simulink model "CrazyClover_angular_velocity_control_PID"  (R2020b)
settings: Solver=VariableStepAuto  StartTime=0.0  StopTime=0.1  RelTol=1e-3
libraries: pid_lib x1
settings Model: Creator=kt012  LastModifiedBy=kt012

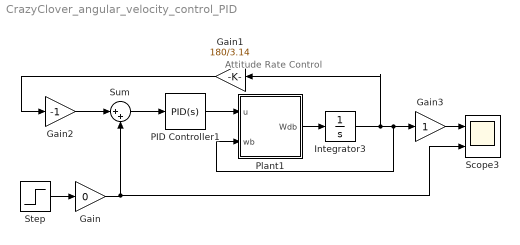
== system CrazyClover_angular_velocity_control_PID ==
  note: Attitude Rate Control
  Gain : Gain  Gain=0
  Gain1 : Gain  Gain=180/3.14
  Gain2 : Gain  Gain=-1
  Gain3 : Gain
  Integrator3 : Integrator  InitialCondition=[1 0 0];  ContinuousStateAttributes='Wb'
  PID Controller1 : pid_lib/PID Controller  Controller=PID  Form=Parallel  TimeDomain=Continuous-time  UseExternalTs=off  SampleTime=-1  IntegratorMethod=Forward Euler  FilterMethod=Forward Euler  ControllerParametersSource=internal  P=50  I=50  D=0  UseFilter=on  N=100  TunerSelectOption=Transfer Function Based (PID Tuner App)  InitialConditionSource=internal  InitialConditionForIntegrator=0  InitialConditionForFilter=0  DifferentiatorICPrevScaledInput=0  ExternalReset=none  TrackingMode=off  Kt=1  LimitOutput=off  SatLimitsSource=internal  UpperSaturationLimit=inf  LowerSaturationLimit=-inf  LinearizeAsGain=on  AntiWindupMode=none  Kb=1  POutMin=[]  POutMax=[]  IOutMin=[]  IOutMax=[]  DOutMin=[]  DOutMax=[]  NOutMin=[]  NOutMax=[]  SumOutMin=[]  SumOutMax=[]  SaturationOutMin=[]  SaturationOutMax=[]  PParamMin=[]  PParamMax=[]  IParamMin=[]  IParamMax=[]  DParamMin=[]  DParamMax=[]  NParamMin=[]  NParamMax=[]  KbParamMin=[]  KbParamMax=[]  KtParamMin=[]  KtParamMax=[]  KbOutMin=[]  KbOutMax=[]  KtOutMin=[]  KtOutMax=[]  IntegratorOutMin=[]  IntegratorOutMax=[]  FilterOutMin=[]  FilterOutMax=[]  SumI1OutMin=[]  SumI1OutMax=[]  SumI2OutMin=[]  SumI2OutMax=[]  SumI3OutMin=[]  SumI3OutMax=[]  SumI4OutMin=[]  SumI4OutMax=[]  SumDOutMin=[]  SumDOutMax=[]  DifferentiatorOutMin=[]  DifferentiatorOutMax=[]  FilterDiffOutCoefMin=[]  FilterDiffOutCoefMax=[]  ReciprocalOutMin=[]  ReciprocalOutMax=[]  SumDenOutMin=[]  SumDenOutMax=[]  SumNumOutMin=[]  SumNumOutMax=[]  DivideOutMin=[]  DivideOutMax=[]  UdiffTsProdOutMin=[]  UdiffTsProdOutMax=[]  NTsProdOutMin=[]  NTsProdOutMax=[]  UintegralTsProdOutMin=[]  UintegralTsProdOutMax=[]  UngainTsProdOutMin=[]  UngainTsProdOutMax=[]  IntegratorContinuousStateAttributes=''  IntegratorStateMustResolveToSignalObject=off  IntegratorRTWStateStorageClass=Auto  FilterContinuousStateAttributes=''  FilterStateMustResolveToSignalObject=off  FilterRTWStateStorageClass=Auto  ParallelPVariant=InternalParameters  IdealPVariant=Disabled  IVariant=InternalParameters  DVariant=InternalParameters  IntegratorVariant=Continuous  SatVariant=Disabled  AWVariant=Passthrough  PCopyVariant=Disabled  TRVariant=Disabled  FdbkBlocksVariant=Forward  IdealPFdbkVariant=Disabled  SatFdbkVariant=Disabled  DerivativeFilterVariant=ContFilter  NVariant=InternalParameters  NCopyVariant=Disabled  FilterICVariant=InternalICsFilter  IntegratorICVariant=InternalICs  ExternalResetVariant=Disabled  TRSumVariant=Passthrough  SumFdbkVariant=Disabled  SumVariant=Sum_PID  TsampFilterVariant=InternalTs  TsampNgainVariant=Passthrough  TsampIntegralVariant=Passthrough  ExternalSaturationOutDataTypeStr=Inherit: Same as second input
  Plant1 : Subsystem
  Scope3 : Scope  NumInputPorts=2
  Step : Step  Time=0.5  After=[1 0 0];  SampleTime=0
  Sum : Sum  Inputs=|++
  wires:
  PID Controller1/1 -> Plant1/1(u)
  Plant1/1(Wdb) -> Integrator3/1
  Sum/1 -> PID Controller1/1
  Gain2/1 -> Sum/1
  Integrator3/1 -> Gain1/1, Plant1/2(wb), Gain3/1
  Gain1/1 -> Gain2/1
  Step/1 -> Gain/1
  Gain3/1 -> Scope3/1
  Gain/1 -> Scope3/2, Sum/2

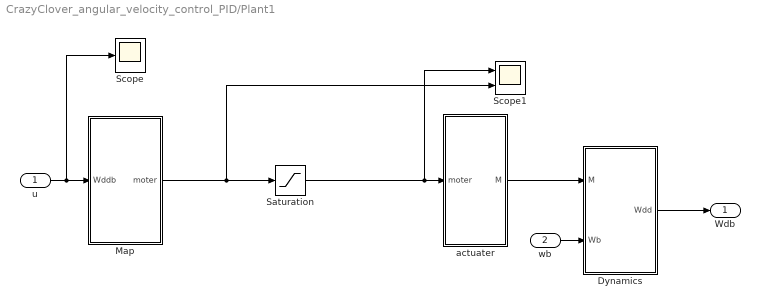
== system CrazyClover_angular_velocity_control_PID/Plant1 ==
  u : Inport
  wb : Inport  Port=2
  Dynamics : MATLAB Function  TreatAsAtomicUnit=on
  Map : MATLAB Function  TreatAsAtomicUnit=on
  Saturation : Saturate  UpperLimit=15000  LowerLimit=-20000
  Scope : Scope
  Scope1 : Scope  NumInputPorts=2
  actuater : MATLAB Function  TreatAsAtomicUnit=on
  Wdb : Outport
  wires:
  wb/1 -> Dynamics/2(Wb)
  actuater/1(M) -> Dynamics/1(M)
  Dynamics/1(Wdd) -> Wdb/1
  u/1 -> Scope/1, Map/1(Wddb)
  Map/1(moter) -> Scope1/2, Saturation/1
  Saturation/1 -> Scope1/1, actuater/1(moter)

== matlab function CrazyClover_angular_velocity_control_PID/Plant1/Map ==
  data: Wddb input; moter output
function moter = fcn(Wddb)


% F [16bit] Wddb [16bit]
maxpwm = 2^14.5;

r = Wddb(1)/2;
p = Wddb(2)/2;
y = Wddb(3);

m1 = - r - p + y;
m2 = - r + p - y;
m3 = + r + p + y;
m4 = + r - p - y;

moter = [m1 m2 m3 m4];
% formation +
% r = min(max(-32000, Wddb(1)), 32000);
% p = min(max(-32000, Wddb(2)), 32000);
% y = min(max(-32000, Wddb(3)), 32000);
% m1 = min(max(0, + p + y), 2^16);
% m2 = min(max(0, - r - y), 2^16);
% m3 = min(max(0, - p + y), 2^16);
% m4 = min(max(0, + r - y), 2^16);

%         ^y
%         |
%         |
%   m3          m4
%
%                    ------>x
%
%   m2          m1

== matlab function CrazyClover_angular_velocity_control_PID/Plant1/actuater ==
  data: moter input; M output
function M = func(moter)

% F [16bit] Wddb [16bit]
m1 = moter(1);
m2 = moter(2);
m3 = moter(3);
m4 = moter(4);
g = 9.8;
Armlength = 0.565/2;
m1 = [2.0775e-07 0.0021 0] * [m1^2;m1;1];
m2 = [2.1910e-07 0.0022 0]  * [m2^2;m2;1];
m3 = [2.1161e-07 0.0024 0]  * [m3^2;m3;1];
m4 = [2.0210e-07 0.0024 0] * [m4^2;m4;1];

% formation X
M1 = Armlength / sqrt(2) * (m3 + m4 - m1 - m2);
M2 = -Armlength / sqrt(2) * (-m3 - m2 + m1 + m4);

% formation + 
% M1 = Armlength  * (m4 - m2);
% M2 = Armlength * (m1 - m3);

M3 = m1 + m3 - m2 - m4;
M = [M1 M2 M3]';

== matlab function CrazyClover_angular_velocity_control_PID/Plant1/Dynamics ==
  data: M input; Wb input; Wdd output
function Wdd = fcn(M,Wb)

% % crazyflie
I = [1 0 0;
     0 1 0;
     0 0 1] * 10^(-2);
% 各加速度計算（ボディー座標系）
Wdd = pinv(I)*(M - cross(Wb, I * Wb));
